simulink model "admittance_control"  (R2026a)
settings: Solver=ode4  StopTime=10  FixedStep=0.001
settings Model: Creator=lhz  LastModifiedBy=lhz

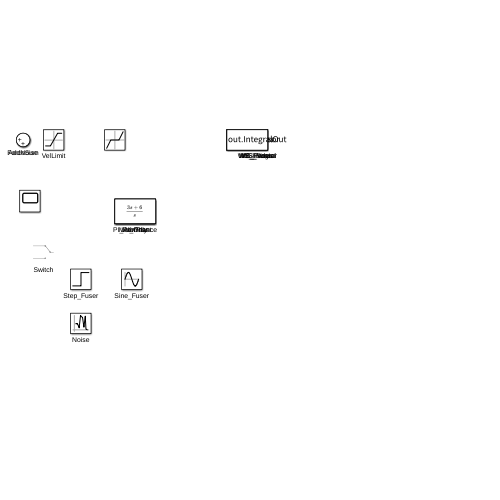
[thumbnail: Simulink's stored preview of the top-level diagram]
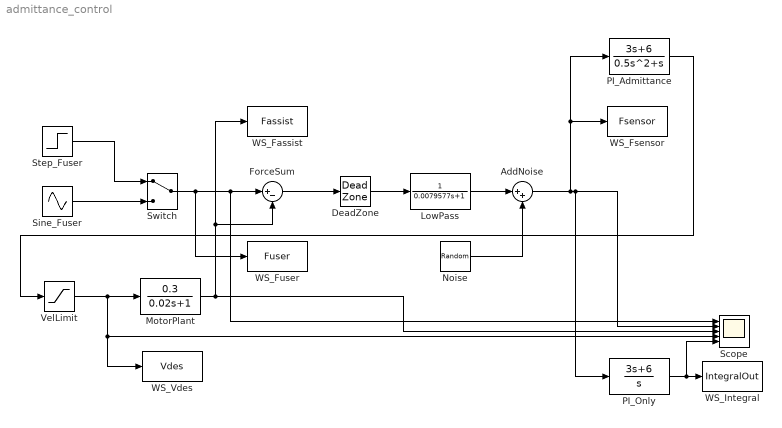
== system admittance_control ==
  AddNoise : Sum  Inputs=|++
  DeadZone : DeadZone  LowerValue=-0.15  UpperValue=0.15
  ForceSum : Sum  Inputs=|+-
  LowPass : TransferFcn  Denominator=[0.0079577 1]
  MotorPlant : TransferFcn  Numerator=0.3  Denominator=[0.02 1]
  Noise : RandomNumber  Variance=0.0025  Seed=42  SampleTime=0.001
  PI_Admittance : TransferFcn  Numerator=[3 6]  Denominator=[0.5 1 0]
  PI_Only : TransferFcn  Numerator=[3 6]  Denominator=[1 0]
  Scope : Scope  NumInputPorts=5
  Sine_Fuser : Sin  Amplitude=5  Frequency=3.1416  SampleTime=0
  Step_Fuser : Step  Time=0.5  FinalValue=10  SampleTime=0
  Switch : ManualSwitch
  VelLimit : Saturate  UpperLimit=300  LowerLimit=-300
  WS_Fassist : ToWorkspace  VariableName=Fassist  SampleTime=-1
  WS_Fsensor : ToWorkspace  VariableName=Fsensor  SampleTime=-1
  WS_Fuser : ToWorkspace  VariableName=Fuser  SampleTime=-1
  WS_Integral : ToWorkspace  VariableName=IntegralOut  SampleTime=-1
  WS_Vdes : ToWorkspace  VariableName=Vdes  SampleTime=-1
  wires:
  PI_Only/1 -> WS_Integral/1, Scope/5
  PI_Admittance/1 -> VelLimit/1
  Noise/1 -> AddNoise/2
  DeadZone/1 -> LowPass/1
  AddNoise/1 -> PI_Only/1, Scope/2, WS_Fsensor/1, PI_Admittance/1
  ForceSum/1 -> DeadZone/1
  MotorPlant/1 -> WS_Fassist/1, ForceSum/2, Scope/3
  Switch/1 -> ForceSum/1, Scope/1, WS_Fuser/1
  LowPass/1 -> AddNoise/1
  VelLimit/1 -> WS_Vdes/1, Scope/4, MotorPlant/1
  Sine_Fuser/1 -> Switch/2
  Step_Fuser/1 -> Switch/1
